simulink model "simulazione"  (R2021a)
settings: Solver=FixedStepAuto  StartTime=0.0  StopTime=20  FixedStep=0.01  RelTol=1e-3
model workspace (MAT data in the model file):
  T = 1
values from neighbouring files (symbols this model uses):
  C_gr = 1029*280    (= 288120)    [parametri_prj.m]
  k_con = 12*280    (= 3360)    [parametri_prj.m]
  Ki_inv = Kp_inv/Ti_inv    [hydroponic_project.m]
  Kp_inv = Mg*sin(phig)/wg    [hydroponic_project.m]
  T_b = 291.15    [parametri_prj.m]
settings Model: Creator=marinacoscione  LastModifiedBy=marinacoscione

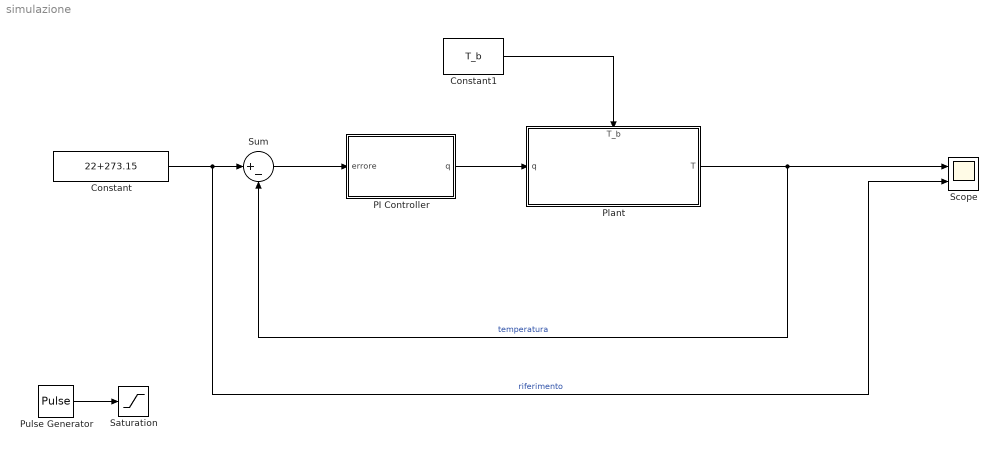
== system simulazione ==
  Constant : Constant  Value=22+273.15
  Constant1 : Constant  Value=T_b
  PI Controller : Subsystem
  Plant : Subsystem
      settings: PortSchema="{\"entries\":[{\"content\":{\"sides\":[{\"content\":{\"connectorIds\":[\"In1\"]},\"type\":\"ConnectorPlacement.EquallySpacedRectSide\",\"uuid\":\"0c3fb8e4-23a3-4b42-a5af-f1c5b75aed2a\"},{\"content\":{\"connectorIds\":[\"Out1\"],\"side\":\"RIGHT\"},\"type\":\"ConnectorPlacement.EquallySpacedRectSide\",\"uuid\":\"ee5652d8-4921-4ea6-bfbc-92dd7bf26615\"},{\"content\":{\"connectorIds\":[\"In2\"],\"side\":\"TOP\"},\"type\":\"ConnectorPlacement.EquallySpacedRectSide\",\"uuid\":\"74fdaef9-ceb7-4d52-aef4-74e0e91fa3dc\"}]},\"type\":\"ConnectorPlacement.EquallySpacedConnector\",\"uuid\":\"eda1a5e3-599e-4b89-bb28-f21db9652c8d\"}],\"packageUris\":[\"http://schema.mathworks.com/mf0/Connector/R2020b\"],\"version\":\"1.0\"}"
  Pulse Generator : DiscretePulseGenerator  PulseType=Time based  Amplitude=22+273.15  Period=8  PulseWidth=50
  Saturation : Saturate  UpperLimit=Inf  LowerLimit=273+16
  Scope : Scope  NumInputPorts=2
  Sum : Sum  Inputs=|+-
  wires:
  Sum/1 -> PI Controller/1(errore)
  PI Controller/1(q) -> Plant/1(q)
  Constant1/1 -> Plant/2(T_b)
  Plant/1(T) -> Sum/2, Scope/1  "temperatura"
  Pulse Generator/1 -> Saturation/1
  Constant/1 -> Scope/2, Sum/1  "riferimento"

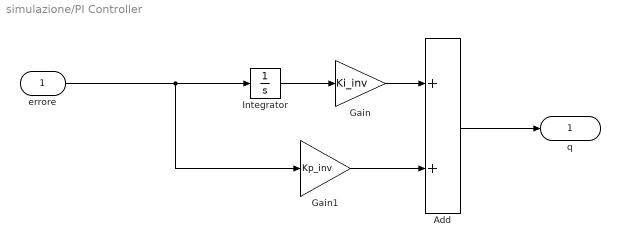
== system simulazione/PI Controller ==
  errore : Inport
  Add : Sum
  Gain : Gain  Gain=Ki_inv
  Gain1 : Gain  Gain=Kp_inv
  Integrator : Integrator
  q : Outport
  wires:
  Gain/1 -> Add/1
  Add/1 -> q/1
  Integrator/1 -> Gain/1
  Gain1/1 -> Add/2
  errore/1 -> Integrator/1, Gain1/1

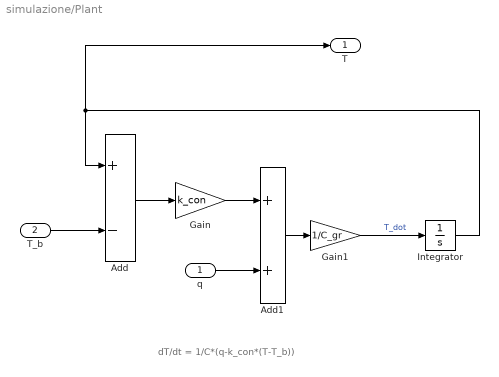
== system simulazione/Plant ==
  note: dT/dt = 1/C*(q-k_con*(T-T_b))
  q : Inport
  T_b : Inport  Port=2
  Add : Sum  Inputs=+-
  Add1 : Sum
  Gain : Gain  Gain=k_con
  Gain1 : Gain  Gain=1/C_gr
  Integrator : Integrator
  T : Outport
  wires:
  Gain1/1 -> Integrator/1  "T_dot"
  Gain/1 -> Add1/1
  q/1 -> Add1/2
  Integrator/1 -> Add/1, T/1
  Add1/1 -> Gain1/1
  Add/1 -> Gain/1
  T_b/1 -> Add/2
